simulink model "untitled"  (R2017b)
settings: Solver=VariableStepAuto  StartTime=0.0  StopTime=30  RelTol=1e-3
undefined symbols (not defined in the file or in its folder): A, B, C, D
settings Model: Creator=Helexium  LastModifiedBy=Helexium

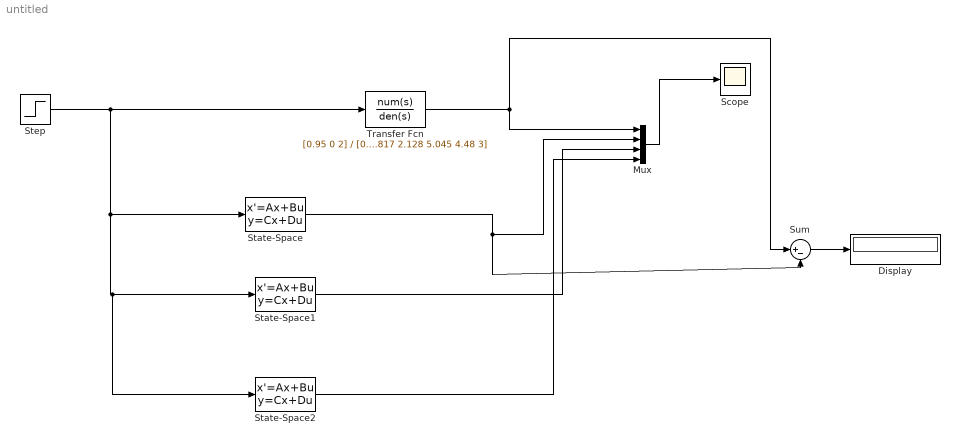
== system untitled ==
  Display : Display
  Mux : Mux
  Scope : Scope
  State-Space : StateSpace  A=A  B=B  C=C  D=D  InitialCondition=0
  State-Space1 : StateSpace  A=A  B=B  C=C  D=D  InitialCondition=[0.5;1;0.5;-1]
  State-Space2 : StateSpace  A=A  B=B  C=C  D=D  InitialCondition=[5,6,3,4]
  Step : Step  SampleTime=0
  Sum : Sum  Inputs=|+-
  Transfer Fcn : TransferFcn  Numerator=[0.95 0 2]  Denominator=[0.817 2.128 5.045 4.48 3]
  wires:
  Step/1 -> Transfer Fcn/1, State-Space2/1, State-Space1/1, State-Space/1
  Transfer Fcn/1 -> Sum/1, Mux/1
  State-Space/1 -> Sum/2, Mux/2
  Mux/1 -> Scope/1
  Sum/1 -> Display/1
  State-Space1/1 -> Mux/3
  State-Space2/1 -> Mux/4
